simulink model "MSFartoystyring"  (R2017b)
settings: Solver=ode45  StartTime=tstart  StopTime=tstop  RelTol=1e-3  EnableMultiTasking=on
values from neighbouring files (symbols this model uses):
  c = 1    [run_task_18.m]
  Kd_r = 1000    [run_task_18.m]
  Ki_u = 1    [run_task_18.m]
  Kp_psi = 10    [run_task_18.m]
  Kp_u = 100    [run_task_18.m]
  nc_max = 85 * 2 * pi / 60    (= 8.90117918517)    [run_task_18.m]
  p0 = zeros(2,1)    [run_task_18.m]
  psi0 = 0    [run_task_18.m]
  r0 = 0    [run_task_18.m]
  tsamp = 10    [run_task_18.m]
  u_d = 7    [run_task_18.m]
  v0 = [0.01 0]'    [run_task_18.m]
undefined symbols (not defined in the file or in its folder): msfartoystyring
settings Model: ExtModeAutoUpdateStatusClock=off  Creator=christh  LastModifiedBy=Ultrawack
settings DataIOCC: LimitDataPoints=on  SaveFormat=Array  SignalLoggingSaveFormat=ModelDataLogs
settings OptimizationCC: ExpressionDepthLimit=2147483647  InitFltsAndDblsToZero=on  LifeSpan=inf
settings DebuggingCC: UnderspecifiedInitializationDetection=Classic  MergeDetectMultiDrivingBlocksExec=none  SolverPrmCheckMsg=warning  FcnCallInpInsideContextMsg=warning  StateNameClashWarn=warning  SFUnexpectedBacktrackingDiag=warning  SFNoUnconditionalDefaultTransitionDiag=warning  SFExecutionAtInitializationDiag=none
settings HardwareCC: ProdBitPerPointer=32  ProdBitPerSizeT=32  ProdBitPerPtrDiffT=32  ProdLargestAtomicFloat=None  ProdIntDivRoundTo=Undefined  ProdEndianess=Unspecified  ProdWordSize=32  ProdHWDeviceType=32-bit Generic
settings ModelReferenceCC: PropagateSignalLabelsOutOfModel=off
settings CodeAppCC: StateflowObjectComments=on
settings GRTTargetCC: TargetLangStandard=C89/C90 (ANSI)  GeneratePreprocessorConditionals=Disable all  CombineOutputUpdateFcns=off  GRTInterface=on
settings ConfigComp: CovMetricSettings=dw  CovHtmlReporting=on  CovSaveCumulativeToWorkspaceVar=on  CovSaveSingleToWorkspaceVar=on  CovExternalEMLEnable=off

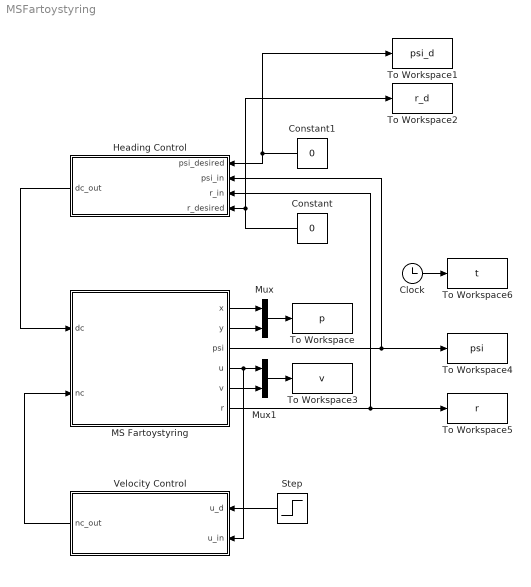
== system MSFartoystyring ==
  Clock : Clock
  Constant : Constant  Value=0
  Constant1 : Constant  Value=0
  Heading Control : Subsystem
  MS Fartoystyring : Subsystem  mask(MS Fartoystyring for Assignment 3 G&C){x0=p0(1), y0=p0(2), u0=v0(1), v0=v0(2), psi0=psi0, r0=r0, c=c}
      mask prompts: x0 "x(t0) (m)"; y0 "y(t0) (m)"; u0 "u(t0) (m/s)"; v0 "v(t0) (m/s)"; psi0 "psi(t0) (rad)"; r0 "r(t0) (rad/s)"; c "current (0 or 1)"
      mask help:
      | Block corresponding to Figure 1 in the assignment text. Gives the response of the ship.
      |
      | The design speed of MS Fartoystyring is u=8.23 m/s.
      |
      | Input:
      | dc: commanded rudder (rad), dmax=25*pi/180
      | nc: commanded shaft speed (rad/s), nmax=85*2*pi/60
      |
      | Output:
      | x: north pos (m)
      | y: east pos (m)
      | u: surge (m/s)
      | v: sway (m/s)
      | psi: heading (rad)
      | r: yaw (rad/s)
      mask Help: Comments, bugs and help requests can be directed to the TA. Email on course website.
  Mux : Mux  Inputs=2
  Mux1 : Mux  Inputs=2
  Step : Step  Time=500  Before=4  After=u_d  SampleTime=0
  To Workspace : ToWorkspace  VariableName=p  SampleTime=tsamp
  To Workspace1 : ToWorkspace  VariableName=psi_d  SampleTime=tsamp
  To Workspace2 : ToWorkspace  VariableName=r_d  SampleTime=tsamp
  To Workspace3 : ToWorkspace  VariableName=v  SampleTime=tsamp
  To Workspace4 : ToWorkspace  VariableName=psi  SampleTime=tsamp
  To Workspace5 : ToWorkspace  VariableName=r  SampleTime=tsamp
  To Workspace6 : ToWorkspace  VariableName=t  SampleTime=tsamp
  Velocity Control : Subsystem
  wires:
  Clock/1 -> To Workspace6/1
  MS Fartoystyring/1(x) -> Mux/1
  MS Fartoystyring/2(y) -> Mux/2
  MS Fartoystyring/5(v) -> Mux1/2
  Mux/1 -> To Workspace/1
  Mux1/1 -> To Workspace3/1
  MS Fartoystyring/3(psi) -> Heading Control/2(psi_in), To Workspace4/1
  MS Fartoystyring/6(r) -> Heading Control/3(r_in), To Workspace5/1
  Heading Control/1(dc_out) -> MS Fartoystyring/1(dc)
  Constant1/1 -> Heading Control/1(psi_desired), To Workspace1/1
  Constant/1 -> To Workspace2/1, Heading Control/4(r_desired)
  Step/1 -> Velocity Control/1(u_d)
  MS Fartoystyring/4(u) -> Velocity Control/2(u_in), Mux1/1
  Velocity Control/1(nc_out) -> MS Fartoystyring/2(nc)

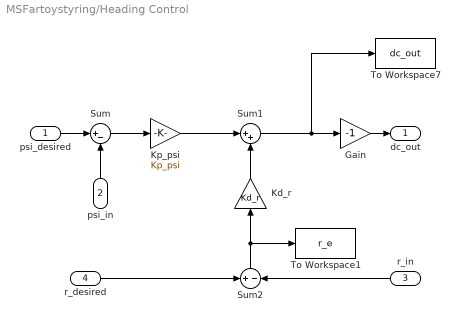
== system MSFartoystyring/Heading Control ==
  psi_desired : Inport
  psi_in : Inport  Port=2
  r_in : Inport  Port=3
  r_desired : Inport  Port=4
  Gain : Gain  Gain=-1
  Kd_r : Gain  Gain=Kd_r
  Kp_psi : Gain  Gain=Kp_psi
  Sum : Sum  Inputs=|+-
  Sum1 : Sum  Inputs=|++
  Sum2 : Sum  Inputs=+|-
  To Workspace1 : ToWorkspace  VariableName=r_e  SampleTime=tsamp
  To Workspace7 : ToWorkspace  VariableName=dc_out  SampleTime=tsamp
  dc_out : Outport
  wires:
  Sum1/1 -> To Workspace7/1, Gain/1
  psi_desired/1 -> Sum/1
  psi_in/1 -> Sum/2
  Sum/1 -> Kp_psi/1
  Gain/1 -> dc_out/1
  r_desired/1 -> Sum2/1
  r_in/1 -> Sum2/2
  Sum2/1 -> To Workspace1/1, Kd_r/1
  Kp_psi/1 -> Sum1/1
  Kd_r/1 -> Sum1/2

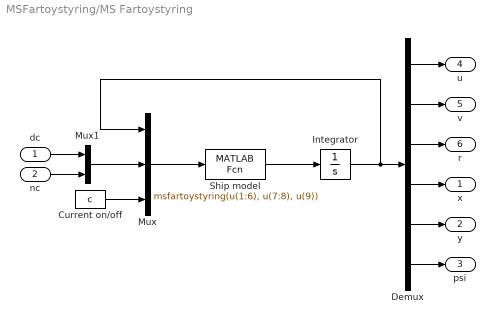
== system MSFartoystyring/MS Fartoystyring ==
  dc : Inport
  nc : Inport  Port=2
  Current on/off : Constant  Value=c
  Demux : Demux  Outputs=6
  Integrator : Integrator  InitialCondition=[u0 v0 r0 x0 y0 psi0]'
  Mux : Mux  Inputs=3
  Mux1 : Mux  Inputs=2
  Ship model : MATLABFcn  MATLABFcn=msfartoystyring(u(1:6), u(7:8), u(9))  OutputDimensions=6
  x : Outport
  y : Outport  Port=2
  psi : Outport  Port=3
  u : Outport  Port=4
  v : Outport  Port=5
  r : Outport  Port=6
  wires:
  Integrator/1 -> Mux/1, Demux/1
  Mux1/1 -> Mux/2
  dc/1 -> Mux1/1
  nc/1 -> Mux1/2
  Demux/1 -> u/1
  Demux/2 -> v/1
  Demux/3 -> r/1
  Demux/4 -> x/1
  Demux/5 -> y/1
  Demux/6 -> psi/1
  Current on/off/1 -> Mux/3
  Ship model/1 -> Integrator/1
  Mux/1 -> Ship model/1

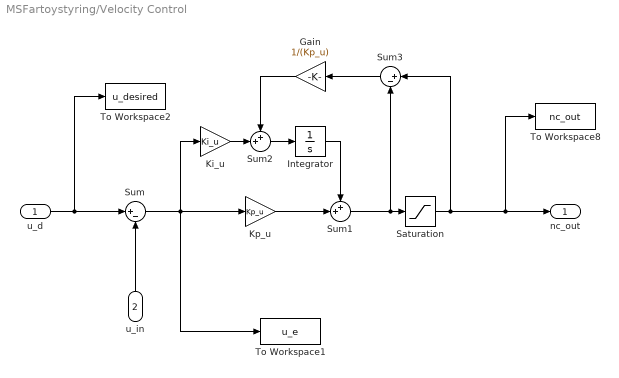
== system MSFartoystyring/Velocity Control ==
  u_d : Inport
  u_in : Inport  Port=2
  Gain : Gain  Gain=1/(Kp_u)
  Integrator : Integrator
  Ki_u : Gain  Gain=Ki_u
  Kp_u : Gain  Gain=Kp_u
  Saturation : Saturate  UpperLimit=nc_max  LowerLimit=-nc_max
  Sum : Sum  Inputs=|+-
  Sum1 : Sum  Inputs=++|
  Sum2 : Sum  Inputs=++|
  Sum3 : Sum  Inputs=|+-
  To Workspace1 : ToWorkspace  VariableName=u_e  SampleTime=tsamp
  To Workspace2 : ToWorkspace  VariableName=u_desired  SampleTime=tsamp
  To Workspace8 : ToWorkspace  VariableName=nc_out  SampleTime=tsamp
  nc_out : Outport
  wires:
  Sum1/1 -> Sum3/2, Saturation/1
  u_in/1 -> Sum/2
  u_d/1 -> Sum/1, To Workspace2/1
  Kp_u/1 -> Sum1/2
  Sum/1 -> Ki_u/1, To Workspace1/1, Kp_u/1
  Ki_u/1 -> Sum2/2
  Sum2/1 -> Integrator/1
  Integrator/1 -> Sum1/1
  Saturation/1 -> Sum3/1, nc_out/1, To Workspace8/1
  Sum3/1 -> Gain/1
  Gain/1 -> Sum2/1
